simulink model "ProcessFlowRateModel_symbiotic_2014APR18"  (Simulink 7.9)
settings: Solver=VariableStepDiscrete  StartTime=0.0  StopTime=10000  RelTol=1e-3
libraries: simeventslib x9
(part 2 of 2)

== matlab function Subsystem4/Selector Acquire ==
  data: En output double; Carton_Count input double
function En = fcn(Carton_Count)

aVarTruthTableCondition_1 = false;


% New Order

aVarTruthTableCondition_1 = logical(Carton_Count == 0);

if (aVarTruthTableCondition_1)
    aFcnTruthTableAction_1();
else % Default
    aFcnTruthTableAction_2();
end

function aFcnTruthTableAction_1()

% Release Selector

En = 1;

function aFcnTruthTableAction_2()

% Return Selector

En = 0;

== matlab function Subsystem4/Selector Release ==
  data: En output double; Carton_Count input double
function En = fcn(Carton_Count)

aVarTruthTableCondition_1 = false;


% Order fully picked

aVarTruthTableCondition_1 = logical(Carton_Count == 60);

if (aVarTruthTableCondition_1)
    aFcnTruthTableAction_1();
else % Default
    aFcnTruthTableAction_2();
end

function aFcnTruthTableAction_1()

% Release Selector

En = 1;

function aFcnTruthTableAction_2()

% Return Selector

En = 0;

== matlab function Subsystem4/Symbotic Flow ==
  data: Remaining_Cartons input double; En output double; Carton_Count input double; Reset_Count output double; Carton_Qty input double; PopUp_Qty input double
function [En, Reset_Count] = fcn(Remaining_Cartons, Carton_Count, Carton_Qty, PopUp_Qty)

aVarTruthTableCondition_1 = false;
aVarTruthTableCondition_2 = false;


% Order fully picked

aVarTruthTableCondition_1 = logical(Carton_Count == (Carton_Qty-1));

% Accumulator Available

aVarTruthTableCondition_2 = logical(Remaining_Cartons <= PopUp_Qty);

if (aVarTruthTableCondition_1 && aVarTruthTableCondition_2)
    aFcnTruthTableAction_1();
elseif (aVarTruthTableCondition_1 && ~aVarTruthTableCondition_2)
    aFcnTruthTableAction_2();
elseif (~aVarTruthTableCondition_1 && aVarTruthTableCondition_2)
    aFcnTruthTableAction_3();
else % Default
    aFcnTruthTableAction_3();
end

function aFcnTruthTableAction_1()

% Allow accumulator flow
% reset count

En = 1;
Reset_Count = 1;

function aFcnTruthTableAction_2()

% Halt accumulator flow
% Do not reset

En = 0;
Reset_Count = 0;

function aFcnTruthTableAction_3()

% Allow accumulator flow
% Do not reset

En = 1;
Reset_Count = 0;

== matlab function Subsystem5/Selector Acquire ==
  data: En output double; Carton_Count input double
function En = fcn(Carton_Count)

aVarTruthTableCondition_1 = false;


% New Order

aVarTruthTableCondition_1 = logical(Carton_Count == 0);

if (aVarTruthTableCondition_1)
    aFcnTruthTableAction_1();
else % Default
    aFcnTruthTableAction_2();
end

function aFcnTruthTableAction_1()

% Release Selector

En = 1;

function aFcnTruthTableAction_2()

% Return Selector

En = 0;

== matlab function Subsystem5/Selector Release ==
  data: En output double; Carton_Count input double
function En = fcn(Carton_Count)

aVarTruthTableCondition_1 = false;


% Order fully picked

aVarTruthTableCondition_1 = logical(Carton_Count == 60);

if (aVarTruthTableCondition_1)
    aFcnTruthTableAction_1();
else % Default
    aFcnTruthTableAction_2();
end

function aFcnTruthTableAction_1()

% Release Selector

En = 1;

function aFcnTruthTableAction_2()

% Return Selector

En = 0;

== matlab function Subsystem5/Symbotic Flow ==
  data: Remaining_Cartons input double; En output double; Carton_Count input double; Reset_Count output double; Carton_Qty input double; PopUp_Qty input double
function [En, Reset_Count] = fcn(Remaining_Cartons, Carton_Count, Carton_Qty, PopUp_Qty)

aVarTruthTableCondition_1 = false;
aVarTruthTableCondition_2 = false;


% Order fully picked

aVarTruthTableCondition_1 = logical(Carton_Count == (Carton_Qty-1));

% Accumulator Available

aVarTruthTableCondition_2 = logical(Remaining_Cartons <= PopUp_Qty);

if (aVarTruthTableCondition_1 && aVarTruthTableCondition_2)
    aFcnTruthTableAction_1();
elseif (aVarTruthTableCondition_1 && ~aVarTruthTableCondition_2)
    aFcnTruthTableAction_2();
elseif (~aVarTruthTableCondition_1 && aVarTruthTableCondition_2)
    aFcnTruthTableAction_3();
else % Default
    aFcnTruthTableAction_3();
end

function aFcnTruthTableAction_1()

% Allow accumulator flow
% reset count

En = 1;
Reset_Count = 1;

function aFcnTruthTableAction_2()

% Halt accumulator flow
% Do not reset

En = 0;
Reset_Count = 0;

function aFcnTruthTableAction_3()

% Allow accumulator flow
% Do not reset

En = 1;
Reset_Count = 0;
